simulink model "IO334_IO_test"  (R2022b)
settings: Solver=FixedStepAuto  StartTime=0.0  StopTime=Inf  RelTol=1e-3
model workspace (MAT data in the model file):
  sos1 = Simulink.Parameter
  sos1.Value = [1  0  0  1  0  0; 1  0  0  1  0  0; 1  0  0  1  0  0; 1  0  0  1  0  0]
  sos1.DataType = 'double'
  sos1.Complexity = 'real'
  sos1.Dimensions = [4 6]
  sos2 = Simulink.Parameter
  sos2.Value = [0  0  0  1  0  0; 1  0  0  1  0  0; 1  0  0  1  0  0; 1  0  0  1  0  0]
  sos2.DataType = 'double'
  sos2.Complexity = 'real'
  sos2.Dimensions = [4 6]
  stdev = Simulink.Parameter
  stdev.Value = 0.2
  stdev.DataType = 'double'
  stdev.Complexity = 'real'
  stdev.Dimensions = [1 1]
libraries: slrealtimeloglib x2, SG_library x2
settings Model: LastModifiedBy=mavolery
settings SolverCC: ConcurrentTasks=on  PositivePriorityOrder=on
settings OptimizationCC: BlockReduction=off  BooleanDataType=off  DefaultParameterBehavior=Inlined  OptimizeBlockIOStorage=off
settings DebuggingCC: SaveWithParameterizedLinksMsg=none  UnderspecifiedInitializationDetection=Classic  MergeDetectMultiDrivingBlocksExec=none  SignalResolutionControl=TryResolveAllWithWarning  InheritedTsInSrcMsg=none  TasksWithSamePriorityMsg=none
settings HardwareCC: ProdBitPerLong=64  ProdLongLongMode=on  ProdHWDeviceType=Intel->x86-64 (Linux 64)
settings ModelReferenceCC: EnableRefExpFcnMdlSchedulingChecks=on  PropagateSignalLabelsOutOfModel=off
settings RTWCC: Description=Simulink Real-Time  SystemTargetFile=slrealtime.tlc  TemplateMakefile=slrealtime_default_tmf  RTWVerbose=off  Toolchain=Simulink Real-Time Toolchain  BuildConfiguration=Faster Runs  CodeExecutionProfiling=on  TargetLang=C++

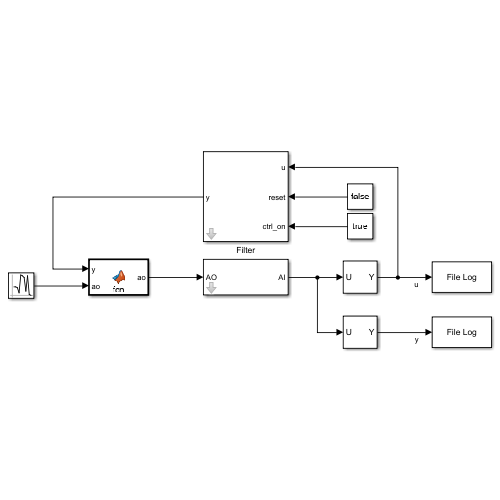
[thumbnail: Simulink's stored preview of the top-level diagram]
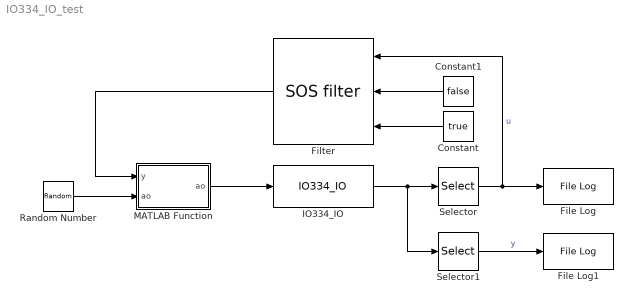
== system IO334_IO_test ==
  Constant : Constant  Value=true  SampleTime=-1
  Constant1 : Constant  Value=false  SampleTime=-1
  File Log : slrealtimeloglib/File Log  decimation=1  inputProcessing=Elements as channels (sample based)
  File Log1 : slrealtimeloglib/File Log  decimation=1  inputProcessing=Elements as channels (sample based)
  Filter : SG_library/Source elements/SOS filter  sos1=sos1  sos2=sos2  limit_ctrl=10  ts=-1
      settings: SourceProductName=Custom Speedgoat implementations
  IO334_IO : SG_library/Built elements/IO334_IO  ts=-1  span=Auto (same as ADC)
      settings: SourceProductName=Custom Speedgoat implementations
  MATLAB Function : MATLAB Function  TreatAsAtomicUnit=on
  Random Number : RandomNumber  Variance=stdev*[0 0 1 1 1 1 1 1 1 1 1 1 1 1 1 1]  Seed=0:15  SampleTime=5e-05
  Selector : Selector  InputPortWidth=16  IndexOptions=Index vector (dialog)  Indices=1:2  OutputSizes=1
  Selector1 : Selector  InputPortWidth=16  IndexOptions=Index vector (dialog)  Indices=3  OutputSizes=1
  wires:
  IO334_IO/1 -> Selector/1, Selector1/1
  Selector1/1 -> File Log1/1  "y"
  Selector/1 -> File Log/1, Filter/1  "u"
  Constant/1 -> Filter/3
  Constant1/1 -> Filter/2
  Random Number/1 -> MATLAB Function/2("ao ")
  MATLAB Function/1(ao) -> IO334_IO/1
  Filter/1 -> MATLAB Function/1(y)

== matlab function IO334_IO_test/MATLAB Function ==
  data: y input; ao output; ao input
function ao = fcn(y, ao)
    ao(1) = y;
end
